simulink model "MTPA_IPMSM"  (R2021b)
settings: Solver=VariableStepAuto  StartTime=0.0  StopTime=0.7  MaxStep=1e-5  RelTol=1e-3
InitFcn:
  | parametrizacija_PMSM
values from neighbouring files (symbols this model uses):
  b_a_MTPA = 2*(alpha_s_MTPA * J_m - b) / (3*p_p^2*psi_r)    [parametrizacija_PMSM.m]
  I_max = 778    [podatki_PMSM.m]
  J_m = 0.003    [podatki_PMSM.m]
  k_id = alpha_c * R_s    [parametrizacija_PMSM.m]
  k_iq = alpha_c * R_s    [parametrizacija_PMSM.m]
  k_is_MTPA = 2*alpha_s_MTPA^2 * J_m / (3*p_p^2*psi_r)    [parametrizacija_PMSM.m]
  k_pd = alpha_c * L_d    [parametrizacija_PMSM.m]
  k_pq = alpha_c * L_q    [parametrizacija_PMSM.m]
  k_ps_MTPA = 2*alpha_s_MTPA * J_m / (3*p_p^2*psi_r)    [parametrizacija_PMSM.m]
  L_d = 0.013e-3    (= 1.3e-05)    [podatki_PMSM.m]
  L_q = 0.029e-3    (= 2.9e-05)    [podatki_PMSM.m]
  M = [0 -1; 1 0]    [parametrizacija_PMSM.m]
  p_p = 4    [podatki_PMSM.m]
  psi_r = 12.1e-3    (= 0.0121)    [podatki_PMSM.m]
  R_s = 3.3e-3    (= 0.0033)    [podatki_PMSM.m]
  T_Z = 1/3 * [2 -1 -1 ... (first row only)    [parametrizacija_PMSM.m]
  U_dc = 48    [podatki_PMSM.m]
  U_s = U_dc/sqrt(3)    [parametrizacija_PMSM.m]
  X = [1/L_d 0 ... (first row only)    [parametrizacija_PMSM.m]
libraries: spsTriangleGeneratorLib x1
settings Model: Creator=Matej  LastModifiedBy=Matej
settings SolverCC: ZeroCrossAlgorithm=Adaptive
settings DebuggingCC: IgnoredZcDiagnostic=none

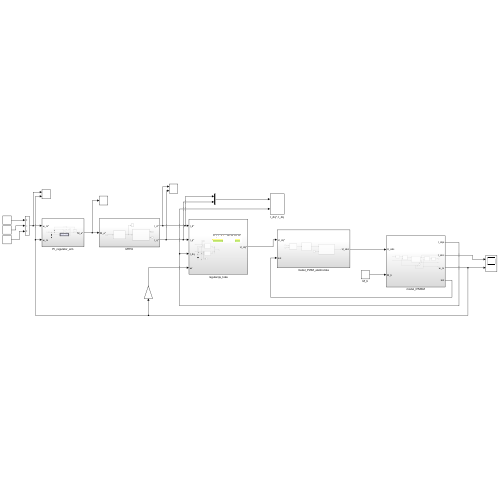
[thumbnail: Simulink's stored preview of the top-level diagram]
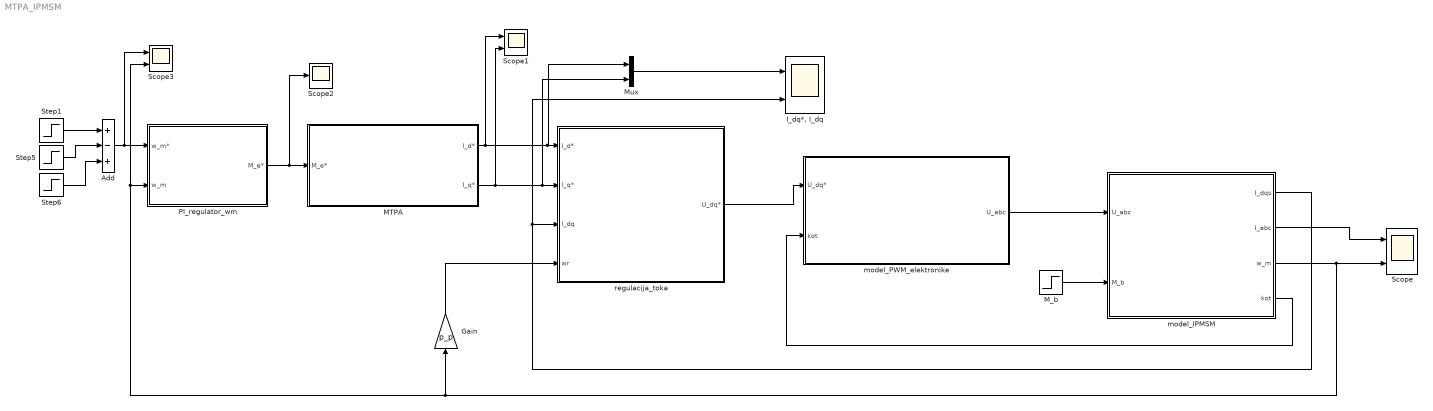
== system MTPA_IPMSM ==
  Add : Sum  Inputs=+-+
  Gain : Gain  Gain=p_p
  "I_dq*, I_dq" : Scope  NumInputPorts=2
  MTPA : Subsystem
  M_b : Step  Time=0.6  After=15  SampleTime=0
  Mux : Mux  Inputs=2
  PI_regulator_wm : Subsystem
  Scope : Scope  NumInputPorts=2
  Scope1 : Scope  NumInputPorts=2
  Scope2 : Scope
  Scope3 : Scope  NumInputPorts=2
  Step1 : Step  Time=0.05  After=400  SampleTime=0
  Step5 : Step  Time=0.15  After=800  SampleTime=0
  Step6 : Step  Time=0.45  After=800  SampleTime=0
  model_IPMSM : Subsystem
  model_PWM_elektronike : Subsystem
  regulacija_toka : Subsystem
  wires:
  model_PWM_elektronike/1(U_abc) -> model_IPMSM/1(U_abc)
  model_IPMSM/4(kot) -> model_PWM_elektronike/2(kot)
  M_b/1 -> model_IPMSM/2(M_b)
  regulacija_toka/1(U_dq*) -> model_PWM_elektronike/1(U_dq*)
  model_IPMSM/1(I_dqs) -> "I_dq*, I_dq"/2, regulacija_toka/3(I_dq)
  MTPA/1(I_d*) -> Scope1/1, Mux/1, regulacija_toka/1(I_d*)
  model_IPMSM/2(I_abc) -> Scope/1
  MTPA/2(I_q*) -> Scope1/2, Mux/2, regulacija_toka/2(I_q*)
  PI_regulator_wm/1(M_e*) -> Scope2/1, MTPA/1(M_e*)
  model_IPMSM/3(w_m) -> Scope3/2, PI_regulator_wm/2(w_m), Gain/1, Scope/2
  Gain/1 -> regulacija_toka/4(wr)
  Mux/1 -> "I_dq*, I_dq"/1
  Add/1 -> Scope3/1, PI_regulator_wm/1(w_m*)
  Step1/1 -> Add/1
  Step5/1 -> Add/2
  Step6/1 -> Add/3

== system MTPA_IPMSM/MTPA ==
  M_e* : Inport
  Scope : Scope
  dolocitev_I_ref : Subsystem
  dolocitev_tokov : Subsystem
  I_d* : Outport
  I_q* : Outport  Port=2
  wires:
  M_e*/1 -> dolocitev_I_ref/1(M*)
  dolocitev_I_ref/1(I_ref*) -> Scope/1, dolocitev_tokov/1(I_ref)
  dolocitev_tokov/2(I_q*) -> I_q*/1
  dolocitev_tokov/1(I_d*) -> I_d*/1

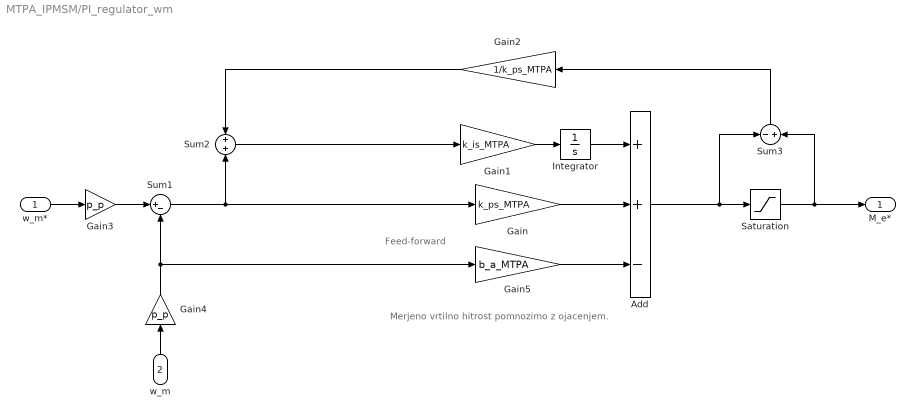
== system MTPA_IPMSM/PI_regulator_wm ==
  note: Merjeno vrtilno hitrost pomnozimo z ojacenjem.
  note: Feed-forward
  w_m* : Inport
  w_m : Inport  Port=2
  Add : Sum  Inputs=++-
  Gain : Gain  Gain=k_ps_MTPA
  Gain1 : Gain  Gain=k_is_MTPA
  Gain2 : Gain  Gain=1/k_ps_MTPA
  Gain3 : Gain  Gain=p_p
  Gain4 : Gain  Gain=p_p
  Gain5 : Gain  Gain=b_a_MTPA
  Integrator : Integrator
  Saturation : Saturate  UpperLimit=56.4828  LowerLimit=-56.4828
  Sum1 : Sum  Inputs=|+-
  Sum2 : Sum
  Sum3 : Sum  Inputs=-+
  M_e* : Outport
  wires:
  w_m/1 -> Gain4/1
  w_m*/1 -> Gain3/1
  Sum1/1 -> Gain/1, Sum2/2
  Gain/1 -> Add/2
  Integrator/1 -> Add/1
  Add/1 -> Sum3/1, Saturation/1
  Saturation/1 -> Sum3/2, M_e*/1
  Gain1/1 -> Integrator/1
  Sum2/1 -> Gain1/1
  Gain3/1 -> Sum1/1
  Gain4/1 -> Sum1/2, Gain5/1
  Gain5/1 -> Add/3
  Gain2/1 -> Sum2/1
  Sum3/1 -> Gain2/1

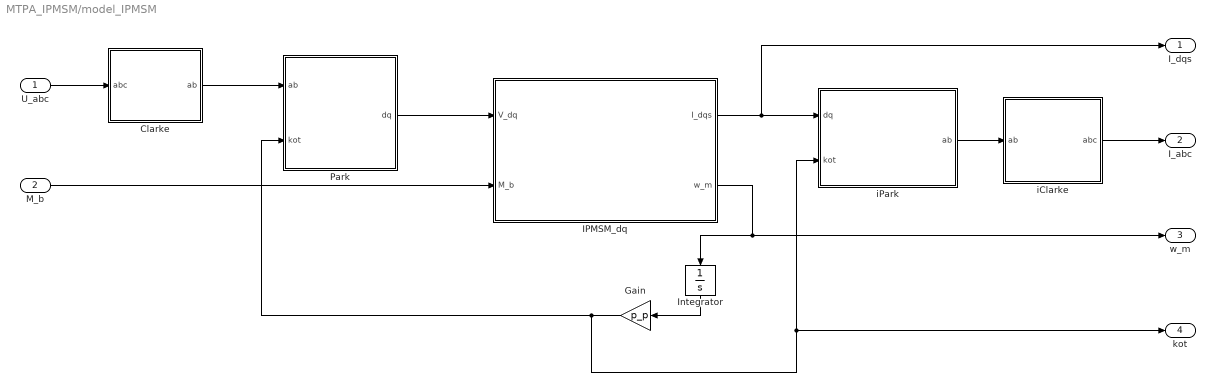
== system MTPA_IPMSM/model_IPMSM ==
  U_abc : Inport
  M_b : Inport  Port=2
  Clarke : Subsystem
  Gain : Gain  Gain=p_p
  IPMSM_dq : Subsystem
  Integrator : Integrator
  Park : Subsystem
  iClarke : Subsystem
  iPark : Subsystem
  I_dqs : Outport
  I_abc : Outport  Port=2
  w_m : Outport  Port=3
  kot : Outport  Port=4
  wires:
  IPMSM_dq/1(I_dqs) -> I_dqs/1, iPark/1(dq)
  U_abc/1 -> Clarke/1(abc)
  Park/1(dq) -> IPMSM_dq/1(V_dq)
  Clarke/1(ab) -> Park/1(ab)
  iPark/1(ab) -> iClarke/1(ab)
  IPMSM_dq/2(w_m) -> w_m/1, Integrator/1
  iClarke/1(abc) -> I_abc/1
  M_b/1 -> IPMSM_dq/2(M_b)
  Integrator/1 -> Gain/1
  Gain/1 -> Park/2(kot), kot/1, iPark/2(kot)

== system MTPA_IPMSM/model_PWM_elektronike ==
  U_dq* : Inport
  kot : Inport  Port=2
  Constant : Constant  Value=U_dc
  iPark : Subsystem
  mocnostni_pretvornik : Subsystem
  simetricna suboscilacijska metoda : Subsystem
  U_abc : Outport
  wires:
  mocnostni_pretvornik/1(U_abc) -> U_abc/1
  Constant/1 -> mocnostni_pretvornik/2(U_dc)
  simetricna suboscilacijska metoda/1(abc) -> mocnostni_pretvornik/1(abc)
  U_dq*/1 -> iPark/1(dq)
  kot/1 -> iPark/2(kot)
  iPark/1(ab) -> simetricna suboscilacijska metoda/1(U_ab_ref)  "U_ab*"

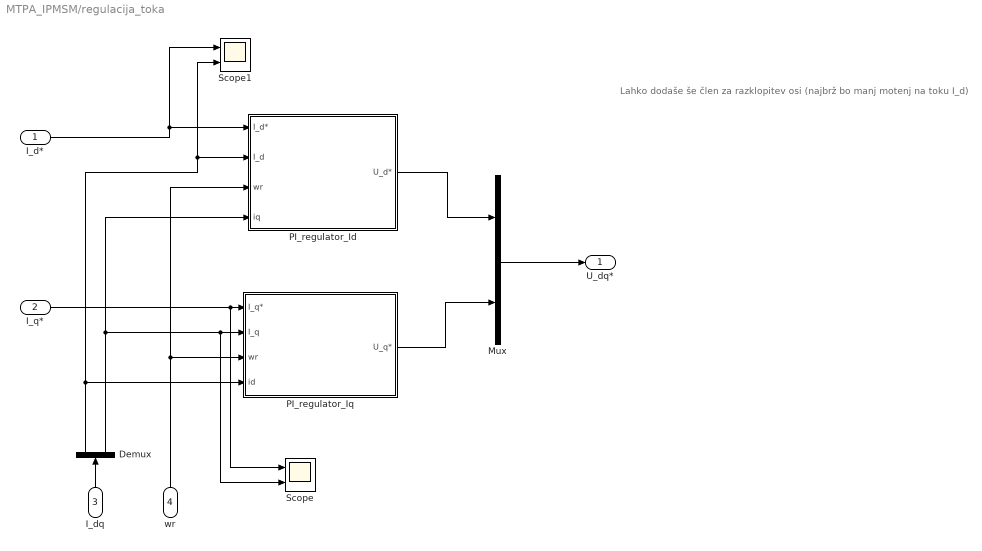
== system MTPA_IPMSM/regulacija_toka ==
  note: Lahko dodaše še člen za razklopitev osi (najbrž bo manj motenj na toku I_d)
  I_d* : Inport
  I_q* : Inport  Port=2
  I_dq : Inport  Port=3
  wr : Inport  Port=4
  Demux : Demux  Outputs=2
  Mux : Mux  Inputs=2
  PI_regulator_Id : Subsystem
  PI_regulator_Iq : Subsystem
  Scope : Scope  NumInputPorts=2
  Scope1 : Scope  NumInputPorts=2
  U_dq* : Outport
  wires:
  I_q*/1 -> Scope/1, PI_regulator_Iq/1(I_q*)
  Mux/1 -> U_dq*/1
  PI_regulator_Iq/1(U_q*) -> Mux/2
  I_dq/1 -> Demux/1
  Demux/2 -> PI_regulator_Id/4(iq), Scope/2, PI_regulator_Iq/2(I_q)
  Demux/1 -> Scope1/2, PI_regulator_Id/2(I_d), PI_regulator_Iq/4(id)
  PI_regulator_Id/1(U_d*) -> Mux/1
  I_d*/1 -> Scope1/1, PI_regulator_Id/1(I_d*)
  wr/1 -> PI_regulator_Id/3(wr), PI_regulator_Iq/3(wr)

== system MTPA_IPMSM/MTPA/dolocitev_I_ref ==
  M* : Inport
  Abs : Abs
  Constant : Constant  Value=I_max
  Gain : Gain  Gain=2/(3*p_p)
  Gain1 : Gain  Gain=1/psi_r
  Max of Elements : MinMax
  Mux : Mux  Inputs=2
  Product : Product
  Sign : Signum
  I_ref* : Outport
  wires:
  Gain/1 -> Gain1/1
  Mux/1 -> Max of Elements/1
  Gain1/1 -> Mux/1
  Constant/1 -> Mux/2
  Abs/1 -> Gain/1
  M*/1 -> Sign/1, Abs/1
  Max of Elements/1 -> Product/2
  Product/1 -> I_ref*/1
  Sign/1 -> Product/1

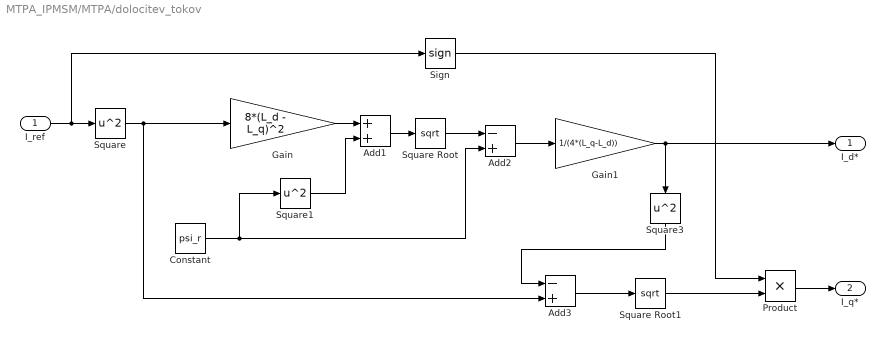
== system MTPA_IPMSM/MTPA/dolocitev_tokov ==
  I_ref : Inport
  Add1 : Sum
  Add2 : Sum  Inputs=-+
  Add3 : Sum  Inputs=-+
  Constant : Constant  Value=psi_r
  Gain : Gain  Gain=8*(L_d - L_q)^2
  Gain1 : Gain  Gain=1/(4*(L_q-L_d))
  Product : Product
  Sign : Signum
  Square : Math  Operator=square  SaturateOnIntegerOverflow=on
  Square Root : Sqrt  SaturateOnIntegerOverflow=on
  Square Root1 : Sqrt  SaturateOnIntegerOverflow=on
  Square1 : Math  Operator=square  SaturateOnIntegerOverflow=on
  Square3 : Math  Operator=square  SaturateOnIntegerOverflow=on
  I_d* : Outport
  I_q* : Outport  Port=2
  wires:
  Add1/1 -> Square Root/1
  Constant/1 -> Square1/1, Add2/2
  Square3/1 -> Add3/1
  Gain/1 -> Add1/1
  I_ref/1 -> Sign/1, Square/1
  Square Root/1 -> Add2/1
  Add3/1 -> Square Root1/1
  Square/1 -> Add3/2, Gain/1
  Add2/1 -> Gain1/1
  Square1/1 -> Add1/2
  Gain1/1 -> I_d*/1, Square3/1
  Square Root1/1 -> Product/2
  Product/1 -> I_q*/1
  Sign/1 -> Product/1

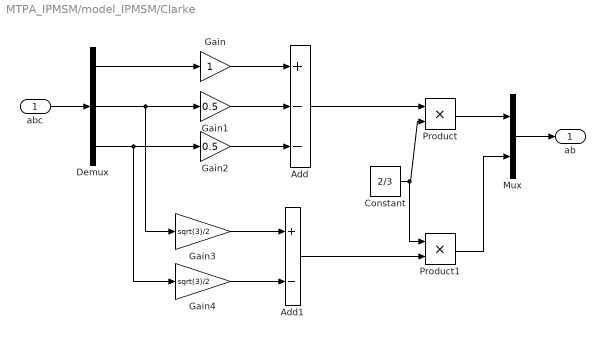
== system MTPA_IPMSM/model_IPMSM/Clarke ==
  abc : Inport
  Add : Sum  Inputs=+--
  Add1 : Sum  Inputs=+-
  Constant : Constant  Value=2/3
  Demux : Demux  Outputs=3
  Gain : Gain
  Gain1 : Gain  Gain=0.5
  Gain2 : Gain  Gain=0.5
  Gain3 : Gain  Gain=sqrt(3)/2
  Gain4 : Gain  Gain=sqrt(3)/2
  Mux : Mux  Inputs=2
  Product : Product
  Product1 : Product
  ab : Outport
  wires:
  Mux/1 -> ab/1
  Demux/2 -> Gain3/1, Gain1/1
  Add/1 -> Product/1
  Demux/3 -> Gain4/1, Gain2/1
  Product/1 -> Mux/1
  Product1/1 -> Mux/2
  Add1/1 -> Product1/2
  Constant/1 -> Product1/1, Product/2
  abc/1 -> Demux/1
  Gain4/1 -> Add1/2
  Demux/1 -> Gain/1
  Gain1/1 -> Add/2
  Gain/1 -> Add/1
  Gain2/1 -> Add/3
  Gain3/1 -> Add1/1

== system MTPA_IPMSM/model_IPMSM/IPMSM_dq ==
  V_dq : Inport
  M_b : Inport  Port=2
  Gain : Gain  Gain=p_p
  M_e : Scope
  Napetostna_enacba : Subsystem
  Navorna_enacba : Subsystem
  Subsystem : Subsystem
  I_dqs : Outport
  w_m : Outport  Port=2
  wires:
  Subsystem/1(w_m) -> w_m/1, Gain/1
  Napetostna_enacba/1(I_dqs) -> I_dqs/1, Navorna_enacba/1(I_dqs)
  V_dq/1 -> Napetostna_enacba/1(V_dq)
  Navorna_enacba/1(M_e) -> M_e/1, Subsystem/1(M_e)
  M_b/1 -> Subsystem/2(M_b)
  Gain/1 -> Napetostna_enacba/2(w_r)

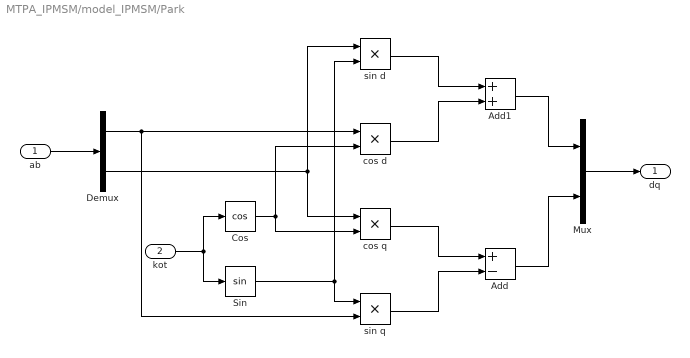
== system MTPA_IPMSM/model_IPMSM/Park ==
  ab : Inport
  kot : Inport  Port=2
  Add : Sum  Inputs=+-
  Add1 : Sum
  Cos : Trigonometry  Operator=cos
  Demux : Demux  Outputs=2
  Mux : Mux  Inputs=2
  Sin : Trigonometry
  cos d : Product
  cos q : Product
  sin d : Product
  sin q : Product
  dq : Outport
  wires:
  Demux/1 -> sin q/2, cos d/1
  Demux/2 -> cos q/1, sin d/1
  sin q/1 -> Add/2
  kot/1 -> Cos/1, Sin/1
  Cos/1 -> cos d/2, cos q/2
  Mux/1 -> dq/1
  Sin/1 -> sin d/2, sin q/1
  cos d/1 -> Add1/2
  cos q/1 -> Add/1
  ab/1 -> Demux/1
  Add1/1 -> Mux/1
  sin d/1 -> Add1/1
  Add/1 -> Mux/2

== system MTPA_IPMSM/model_IPMSM/iClarke ==
  ab : Inport
  Add : Sum  Inputs=-+
  Add1 : Sum  Inputs=--
  Demux : Demux  Outputs=2
  Gain : Gain
  Gain1 : Gain  Gain=0.5
  Gain2 : Gain  Gain=0.5
  Gain3 : Gain  Gain=sqrt(3)/2
  Gain5 : Gain  Gain=sqrt(3)/2
  Mux : Mux  Inputs=3
  abc : Outport
  wires:
  Demux/1 -> Gain2/1, Gain1/1, Gain/1
  Add1/1 -> Mux/3
  Gain3/1 -> Add/2
  Gain2/1 -> Add1/1
  Add/1 -> Mux/2
  Mux/1 -> abc/1
  Gain/1 -> Mux/1
  Demux/2 -> Gain3/1, Gain5/1
  Gain1/1 -> Add/1
  Gain5/1 -> Add1/2
  ab/1 -> Demux/1

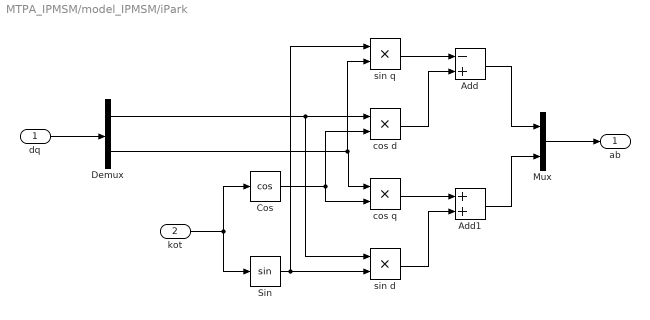
== system MTPA_IPMSM/model_IPMSM/iPark ==
  dq : Inport
  kot : Inport  Port=2
  Add : Sum  Inputs=-+
  Add1 : Sum
  Cos : Trigonometry  Operator=cos
  Demux : Demux  Outputs=2
  Mux : Mux  Inputs=2
  Sin : Trigonometry
  cos d : Product
  cos q : Product
  sin d : Product
  sin q : Product
  ab : Outport
  wires:
  Add/1 -> Mux/1
  Demux/1 -> sin d/1, cos d/1
  Add1/1 -> Mux/2
  Sin/1 -> sin q/1, sin d/2
  dq/1 -> Demux/1
  kot/1 -> Cos/1, Sin/1
  Mux/1 -> ab/1
  sin d/1 -> Add1/2
  Demux/2 -> sin q/2, cos q/1
  Cos/1 -> cos q/2, cos d/2
  cos q/1 -> Add1/1
  cos d/1 -> Add/2
  sin q/1 -> Add/1

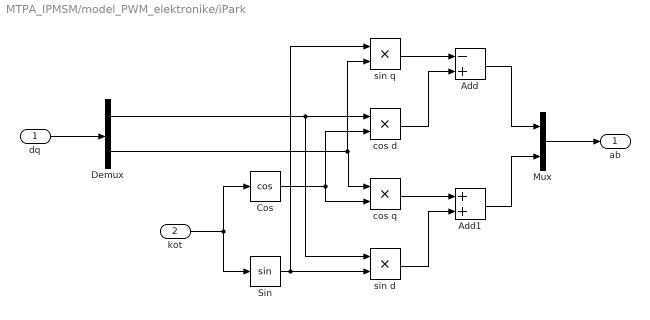
== system MTPA_IPMSM/model_PWM_elektronike/iPark ==
  dq : Inport
  kot : Inport  Port=2
  Add : Sum  Inputs=-+
  Add1 : Sum
  Cos : Trigonometry  Operator=cos
  Demux : Demux  Outputs=2
  Mux : Mux  Inputs=2
  Sin : Trigonometry
  cos d : Product
  cos q : Product
  sin d : Product
  sin q : Product
  ab : Outport
  wires:
  Add/1 -> Mux/1
  Demux/1 -> sin d/1, cos d/1
  Add1/1 -> Mux/2
  Sin/1 -> sin q/1, sin d/2
  dq/1 -> Demux/1
  kot/1 -> Cos/1, Sin/1
  Mux/1 -> ab/1
  sin d/1 -> Add1/2
  Demux/2 -> sin q/2, cos q/1
  Cos/1 -> cos q/2, cos d/2
  cos q/1 -> Add1/1
  cos d/1 -> Add/2
  sin q/1 -> Add/1

== system MTPA_IPMSM/model_PWM_elektronike/mocnostni_pretvornik ==
  abc : Inport
  U_dc : Inport  Port=2
  Demux : Demux  Outputs=3
  Gain : Gain  Gain=1/2
  Gain1 : Gain  Gain=-1/2
  Gain2 : Gain  Gain=T_Z  Multiplication=Matrix(K*u)
  Mux : Mux  Inputs=3
  Switch : Switch  Criteria=u2 > Threshold  Threshold=0.5
  Switch1 : Switch  Criteria=u2 > Threshold  Threshold=0.5
  Switch2 : Switch  Criteria=u2 > Threshold  Threshold=0.5
  U_abc : Outport
  wires:
  abc/1 -> Demux/1
  Switch1/1 -> Mux/2
  Demux/1 -> Switch/2
  Demux/3 -> Switch2/2
  Switch2/1 -> Mux/3
  Gain/1 -> Switch1/1, Switch2/1, Switch/1
  Switch/1 -> Mux/1
  Gain1/1 -> Switch/3, Switch1/3, Switch2/3
  Mux/1 -> Gain2/1
  Gain2/1 -> U_abc/1
  U_dc/1 -> Gain1/1, Gain/1
  Demux/2 -> Switch1/2

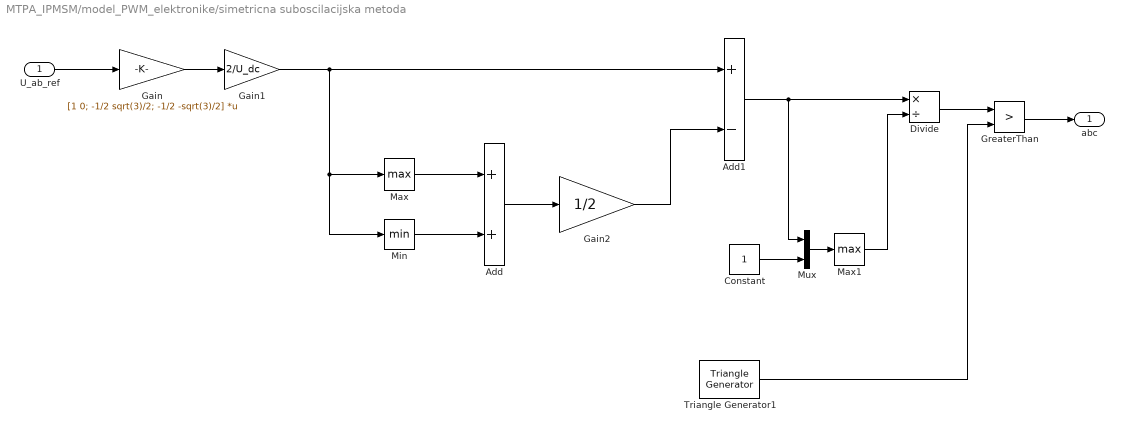
== system MTPA_IPMSM/model_PWM_elektronike/simetricna suboscilacijska metoda ==
  U_ab_ref : Inport
  Add : Sum
  Add1 : Sum  Inputs=+-
  Constant : Constant
  Divide : Product  Inputs=*/
  Gain : Gain  Gain=[1 0; -1/2 sqrt(3)/2; -1/2 -sqrt(3)/2]  Multiplication=Matrix(K*u)
  Gain1 : Gain  Gain=2/U_dc
  Gain2 : Gain  Gain=1/2
  GreaterThan : RelationalOperator  Operator=>  OutDataTypeStr=boolean  RndMeth=Simplest
  Max : MinMax  Function=max
  Max1 : MinMax  Function=max
  Min : MinMax
  Mux : Mux  Inputs=2
  Triangle Generator1 : spsTriangleGeneratorLib/Triangle Generator  Freq=f_sw  Phase=0  Ts=0
  abc : Outport
  wires:
  GreaterThan/1 -> abc/1
  Gain/1 -> Gain1/1
  Add/1 -> Gain2/1
  Max/1 -> Add/1
  Gain2/1 -> Add1/2
  Triangle Generator1/1 -> GreaterThan/2
  U_ab_ref/1 -> Gain/1
  Min/1 -> Add/2
  Gain1/1 -> Max/1, Min/1, Add1/1
  Add1/1 -> Mux/1, Divide/1
  Max1/1 -> Divide/2
  Constant/1 -> Mux/2
  Mux/1 -> Max1/1
  Divide/1 -> GreaterThan/1

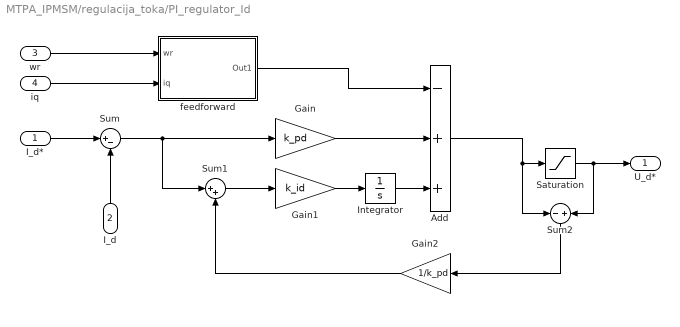
== system MTPA_IPMSM/regulacija_toka/PI_regulator_Id ==
  I_d* : Inport
  I_d : Inport  Port=2
  wr : Inport  Port=3
  iq : Inport  Port=4
  Add : Sum  Inputs=-++
  Gain : Gain  Gain=k_pd
  Gain1 : Gain  Gain=k_id
  Gain2 : Gain  Gain=1/k_pd
  Integrator : Integrator
  Saturation : Saturate  UpperLimit=U_s  LowerLimit=-U_s
  Sum : Sum  Inputs=|+-
  Sum1 : Sum  Inputs=|++
  Sum2 : Sum  Inputs=-+
  feedforward : Subsystem
  U_d* : Outport
  wires:
  I_d*/1 -> Sum/1
  Gain/1 -> Add/2
  Integrator/1 -> Add/3
  Saturation/1 -> Sum2/2, U_d*/1
  Sum/1 -> Sum1/1, Gain/1
  Sum1/1 -> Gain1/1
  Gain2/1 -> Sum1/2
  Add/1 -> Sum2/1, Saturation/1
  Sum2/1 -> Gain2/1
  Gain1/1 -> Integrator/1
  I_d/1 -> Sum/2
  wr/1 -> feedforward/1(wr)
  feedforward/1(Out1) -> Add/1
  iq/1 -> feedforward/2(iq)

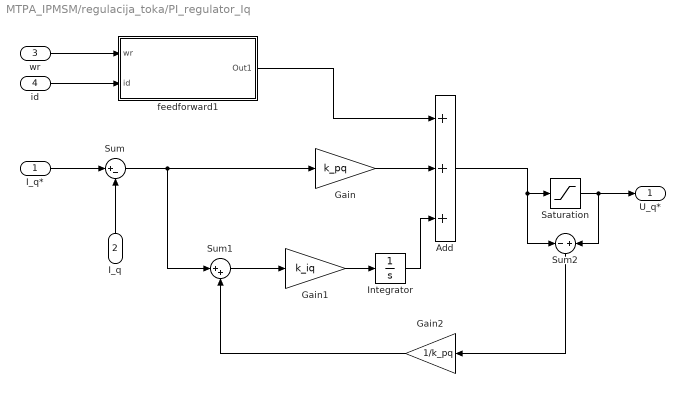
== system MTPA_IPMSM/regulacija_toka/PI_regulator_Iq ==
  I_q* : Inport
  I_q : Inport  Port=2
  wr : Inport  Port=3
  id : Inport  Port=4
  Add : Sum  Inputs=+++
  Gain : Gain  Gain=k_pq
  Gain1 : Gain  Gain=k_iq
  Gain2 : Gain  Gain=1/k_pq
  Integrator : Integrator
  Saturation : Saturate  UpperLimit=U_s  LowerLimit=-U_s
  Sum : Sum  Inputs=|+-
  Sum1 : Sum  Inputs=|++
  Sum2 : Sum  Inputs=-+
  feedforward1 : Subsystem
  U_q* : Outport
  wires:
  I_q/1 -> Sum/2
  Sum/1 -> Sum1/1, Gain/1
  Add/1 -> Sum2/1, Saturation/1
  Saturation/1 -> U_q*/1, Sum2/2
  Gain/1 -> Add/2
  I_q*/1 -> Sum/1
  Gain2/1 -> Sum1/2
  Integrator/1 -> Add/3
  Sum2/1 -> Gain2/1
  Sum1/1 -> Gain1/1
  Gain1/1 -> Integrator/1
  id/1 -> feedforward1/2(id)
  wr/1 -> feedforward1/1(wr)
  feedforward1/1(Out1) -> Add/1

== system MTPA_IPMSM/model_IPMSM/IPMSM_dq/Napetostna_enacba ==
  V_dq : Inport
  w_r : Inport  Port=2
  Add : Sum  Inputs=-+-
  Add1 : Sum  Inputs=+-
  Gain : Gain  Gain=R_s
  Gain1 : Gain  Gain=M  Multiplication=Matrix(K*u)
  Integrator : Integrator
  Product : Product
  mag_fluks_rotorja(TM) : Constant  Value=[psi_r 0]
  matrika induktivnosti : Gain  Gain=X  Multiplication=Matrix(K*u)
  I_dqs : Outport
  wires:
  V_dq/1 -> Add/2
  Add/1 -> Integrator/1
  Gain/1 -> Add/1
  Product/1 -> Add/3
  w_r/1 -> Product/2
  Integrator/1 -> Gain1/1, Add1/1  "psi_dqs"
  Gain1/1 -> Product/1
  mag_fluks_rotorja(TM)/1 -> Add1/2
  Add1/1 -> matrika induktivnosti/1
  matrika induktivnosti/1 -> I_dqs/1, Gain/1

== system MTPA_IPMSM/model_IPMSM/IPMSM_dq/Navorna_enacba ==
  I_dqs : Inport
  Add : Sum
  Demux : Demux  Outputs=2
  Gain : Gain  Gain=3/2*p_p
  Gain1 : Gain  Gain=L_d-L_q
  Gain2 : Gain  Gain=psi_r
  Product : Product
  Scope : Scope  NumInputPorts=2
  Scope1 : Scope  NumInputPorts=2
  M_e : Outport
  wires:
  I_dqs/1 -> Demux/1
  Demux/2 -> Gain2/1, Scope/2, Product/2  "I_qs"
  Product/1 -> Gain1/1
  Demux/1 -> Scope/1, Product/1  "I_ds"
  Add/1 -> Gain/1
  Gain/1 -> M_e/1
  Gain2/1 -> Scope1/2, Add/2
  Gain1/1 -> Scope1/1, Add/1

== system MTPA_IPMSM/model_IPMSM/IPMSM_dq/Subsystem ==
  M_e : Inport
  M_b : Inport  Port=2
  Add : Sum  Inputs=+-
  Gain : Gain  Gain=1/J_m
  Integrator1 : Integrator
  w_m : Outport
  wires:
  Integrator1/1 -> w_m/1
  Add/1 -> Gain/1
  M_b/1 -> Add/2
  Gain/1 -> Integrator1/1
  M_e/1 -> Add/1

== system MTPA_IPMSM/regulacija_toka/PI_regulator_Id/feedforward ==
  wr : Inport
  iq : Inport  Port=2
  Gain3 : Gain  Gain=L_q
  Product : Product
  Out1 : Outport
  wires:
  iq/1 -> Product/2
  Product/1 -> Gain3/1
  Gain3/1 -> Out1/1
  wr/1 -> Product/1

== system MTPA_IPMSM/regulacija_toka/PI_regulator_Iq/feedforward1 ==
  wr : Inport
  id : Inport  Port=2
  Add1 : Sum
  Constant : Constant  Value=psi_r
  Gain3 : Gain  Gain=L_d
  Product : Product
  Product1 : Product
  Out1 : Outport
  wires:
  Gain3/1 -> Add1/2
  id/1 -> Product/2
  Constant/1 -> Product1/1
  Product1/1 -> Add1/1
  Product/1 -> Gain3/1
  Add1/1 -> Out1/1
  wr/1 -> Product/1, Product1/2
